simulink model "CM13_2024a_MachE_for_UA_HIL"  (R2024a)
settings: Solver=ode1  StartTime=0.0  StopTime=Inf  FixedStep=0.001  RelTol=1e-3  EnableMultiTasking=on
PreLoadFcn:
  | % if ~length(which('cmcmd')), cmenv; end
PostLoadFcn:
  | if any(exist('dsrtsu_mdlpostloadfcn', 'file') ~= 0), dsrtsu_mdlpostloadfcn('Execute', bdroot); end
InitFcn:
  | , if any(exist('rtifpga_mdlclblib', 'file') ~= 0), rtifpga_mdlclblib('Init', bdroot); end,
  | , if any(exist('dsmpb_private', 'file') ~= 0), dsmpb_private('dsmpb_mdlclblib', 'Init', bdroot); end,
values from neighbouring files (symbols this model uses):
  CoastDown =     [Run_Simulink.mat]
  limitedMCT =     [Run_Simulink.mat]
  MCT =     [Run_Simulink.mat]
  pMCT =     [Run_Simulink.mat]
  RealSimPara =     [Run_Simulink.mat]
  Ref_speed = [13 13.007895099 13.015778396 13.023649891 13.031509584 13.039357475 13.047193564 13.055017851 13.062830336 13.070631019 13.0784199 13.086196979 ... (2669 elements, 2669x1)]    [Ref_speed_and_time.mat]
  Ref_time = [0 0.01 0.02 0.03 0.04 0.05 0.06 0.07 0.08 0.09 0.1 0.11 ... (2669 elements, 2669x1)]    [Ref_speed_and_time.mat]
  US06 =     [Run_Simulink.mat]
undefined symbols (not defined in the file or in its folder): AccelCmd, ActTqLF_Nm_, ActTqLR_Nm_, ActTqRF_Nm_, ActTqRR_Nm_, BattChargeLimitMaxPwr, BattChargeLimitSocBpts, BattChargeLimitTbl, BattChrgCapcty, BattDischargeLimitSocBpts, BattDischargeLimitTbl, BattDischargeMaxPwr, BattNumCellsParallel, BattNumCellsSeries, BattOpenVoltCapBpts, BattOpenVoltTbl, BattResistSocBpts, BattResistTbl, BattResistTempBpts, BrakeMaxPrs, BrakeMaxTrq, ChassisDistCg2FrontAxle, ChassisDistCg2RearAxle, ChassisVehMass, CltchCmd, DecelCmd, DiffRatio, DiscIntNeverNeededParam, EnvGravCnst, EnvPrs, EnvTemp, FuelSpecificGrav, GearCmd, h, InitStates, lgSw, MtrEffSpdBpts, MtrEffTbl, MtrEffTrqBpts, MtrPwrMax, MtrTrqMax, planned_speed, planned_time, ref_speed, ref_time, rticanmm_blockfcn, rticanmm_initfcn, SteeringCmd, SupvsryCtrlRegenBrkCutOffTbl, SupvsryCtrlRegenSpdBpts, TestScnrioCycleNum, VEH
libraries: simulink x264, VSIGenLib x262, etargetslib x201, dsmpblib x161, CarMaker4SL x142, rtimmsu_dsrtlib x32, vehdynlibtire x24, autolibshared x19, vehdynlibsuspension x14, vehdynlibtirecommon x14, autolibutils x10, VsrLibWheel x8
(part 15 of 48)

== system CM13_2024a_MachE_for_UA_HIL/CarMaker/IPG Vehicle/Rototest and ORNL Interface/Format CM Powertrain Signals ==
  note: Can Bypass with my own brake model
  BrakingTorques : Inport
  RotoWheelSpd : Inport  Port=2
  AxlTrq : Inport  Port=3
  MaxRegen : Inport  Port=4
  Bus Creator1 : BusCreator  Inputs=42
  Bus Selector2 : BusSelector  OutputSignals=Brake IF Trq_WB FL,Brake IF Trq_WB FR,Brake IF Trq_WB RL,Brake IF Trq_WB RR
  BusCreator2 : BusCreator  Inputs=42
  Demux : Demux
  Demux1 : Demux  Outputs=42
      settings: DisplayOption=none
  Demux2 : Demux
  Discrete-Time Integrator{4..7} (4 alike) : DiscreteIntegrator  IntegratorMethod=Integration: Backward Euler  SampleTime=0.001  ICPrevOutput=DiscIntNeverNeededParam  ICPrevScaledInput=DiscIntNeverNeededParam
  Gain{5..8} (4 alike) : Gain  Gain=-1
  Ground{2..5} (4 alike) : Ground
  Ignition : Constant
  Memory{1..4} (4 alike) : Memory
  Operation Error : Constant  Value=4
  Operation State Driving : Constant  Value=4
  Product{1..4} (4 alike) : Product  RndMeth=Zero
  Saturation{1..4} (4 alike) : Saturate  UpperLimit=1  LowerLimit=-1
  Zero{1..5} (5 alike) : Constant  Value=0
  PowerTrainOutIdeal : Outport
  wires:
  Saturation4/1 -> Product4/2
  Demux1/3 -> BusCreator2/3  "PT IF OperationError"
  Demux1/2 -> BusCreator2/2  "PT IF OperationState"
  Demux1/40 -> BusCreator2/40  "PT IF WRR Trq_Supp2WC"
  Demux1/9 -> BusCreator2/9  "PT IF Trq_Supp2Bdy1B x"
  Discrete-Time Integrator6/1 -> Bus Creator1/29  "PT WRL rot"
  Demux1/1 -> BusCreator2/1  "PT IF Ignition"
  MaxRegen/1 -> Bus Creator1/28, Bus Creator1/21
  BusCreator2/1 -> PowerTrainOutIdeal/1
  Operation State Driving/1 -> Bus Creator1/2
  Gain8/1 -> Bus Creator1/38
  Demux1/16 -> BusCreator2/16  "PT IF WFL rotv"
  Demux1/21 -> BusCreator2/21  "PT IF WFL Trq_BrakeReg_max"
  Ground2/1 -> Bus Creator1/7
  Demux1/23 -> BusCreator2/23  "PT IF WFR rotv"
  Demux1/14 -> BusCreator2/14  "PT IF DL_iDiff_mean"
  Demux1/4 -> BusCreator2/4  "PT IF GearNo"
  Demux1/17 -> BusCreator2/17  "PT IF WFL Trq_B2W"
  Product3/1 -> Gain5/1
  Demux1/5 -> BusCreator2/5  "PT IF Engine_rotv"
  Demux1/11 -> BusCreator2/11  "PT IF Trq_Supp2Bdy1B z"
  Demux1/12 -> BusCreator2/12  "PT IF Trq_Supp2BdyEng x"
  Demux1/7 -> BusCreator2/7  "PT IF Trq_Supp2Bdy1 y"
  Discrete-Time Integrator5/1 -> Bus Creator1/22  "PT WFR rot"
  Demux1/42 -> BusCreator2/42  "PT IF WRR Trq_BrakeReg_max"
  Gain5/1 -> Bus Creator1/17
  Demux1/18 -> BusCreator2/18  "PT IF WFL Trq_Drive"
  Demux1/8 -> BusCreator2/8  "PT IF Trq_Supp2Bdy1 z"
  Demux1/38 -> BusCreator2/38  "PT IF WRR Trq_B2W"
  Memory4/1 -> Saturation4/1
  Demux1/10 -> BusCreator2/10  "PT IF Trq_Supp2Bdy1B y"
  Demux1/27 -> BusCreator2/27  "PT IF WFR Trq_BrakeReg"
  Demux1/24 -> BusCreator2/24  "PT IF WFR Trq_B2W"
  Demux1/25 -> BusCreator2/25  "PT IF WFR Trq_Drive"
  Demux1/26 -> BusCreator2/26  "PT IF WFR Trq_Supp2WC"
  Demux1/13 -> BusCreator2/13  "PT IF Trq_Supp2BdyEng y"
  Demux1/15 -> BusCreator2/15  "PT IF WFL rot"
  Bus Selector2/2 -> Product1/1  "<Brake IF Trq_WB FR>"
  Memory3/1 -> Saturation3/1
  Demux1/19 -> BusCreator2/19  "PT IF WFL Trq_Supp2WC"
  Demux1/22 -> BusCreator2/22  "PT IF WFR rot"
  Demux1/29 -> BusCreator2/29  "PT IF WRL rot"
  Demux1/33 -> BusCreator2/33  "PT IF WRL Trq_Supp2WC"
  Demux1/30 -> BusCreator2/30  "PT IF WRL rotv"
  Demux1/28 -> BusCreator2/28  "PT IF WFR Trq_BrakeReg_max"
  Demux1/35 -> BusCreator2/35  "PT IF WRL Trq_BrakeReg_max"
  Demux1/39 -> BusCreator2/39  "PT IF WRR Trq_Drive"
  Zero4/1 -> Bus Creator1/33, Bus Creator1/34, Bus Creator1/35
  Demux1/34 -> BusCreator2/34  "PT IF WRL Trq_BrakeReg"
  Demux1/37 -> BusCreator2/37  "PT IF WRR rotv"
  Demux1/31 -> BusCreator2/31  "PT IF WRL Trq_B2W"
  Demux1/32 -> BusCreator2/32  "PT IF WRL Trq_Drive"
  Demux1/36 -> BusCreator2/36  "PT IF WRR rot"
  Zero3/1 -> Bus Creator1/26, Bus Creator1/27
  Demux/4 -> Memory4/1, Discrete-Time Integrator7/1, Bus Creator1/37  "rotv RR"
  Zero2/1 -> Bus Creator1/19, Bus Creator1/20
  Zero1/1 -> Bus Creator1/5, Bus Creator1/4, Bus Creator1/12, Bus Creator1/14, Bus Creator1/13, Bus Creator1/11, Bus Creator1/10, Bus Creator1/9, Bus Creator1/8
  Demux1/20 -> BusCreator2/20  "PT IF WFL Trq_BrakeReg"
  Product2/1 -> Gain7/1
  Discrete-Time Integrator4/1 -> Bus Creator1/15  "PT WFL rot"
  Demux/2 -> Memory1/1, Discrete-Time Integrator5/1, Bus Creator1/23  "rotv FR"
  Discrete-Time Integrator7/1 -> Bus Creator1/36  "PtT WRR rot"
  Zero5/1 -> Bus Creator1/40, Bus Creator1/41, Bus Creator1/42
  Demux1/6 -> BusCreator2/6  "PT IF Trq_Supp2Bdy1 x"
  Demux1/41 -> BusCreator2/41  "PT IF WRR Trq_BrakeReg"
  BrakingTorques/1 -> Bus Selector2/1
  Operation Error/1 -> Bus Creator1/3
  Demux/3 -> Memory2/1, Discrete-Time Integrator6/1, Bus Creator1/30  "rotv RL"
  Memory1/1 -> Saturation1/1
  Ground4/1 -> Bus Creator1/6
  Bus Selector2/1 -> Product3/1  "<Brake IF Trq_WB FL>"
  Gain6/1 -> Bus Creator1/24
  Ignition/1 -> Bus Creator1/1  "PT Ignition"
  Memory2/1 -> Saturation2/1
  Saturation1/1 -> Product1/2
  Bus Selector2/3 -> Product2/1  "<Brake IF Trq_WB RL>"
  Gain7/1 -> Bus Creator1/31
  Demux/1 -> Memory3/1, Discrete-Time Integrator4/1, Bus Creator1/16  "rotv FL"
  Product4/1 -> Gain8/1
  Bus Creator1/1 -> Demux1/1
  Saturation2/1 -> Product2/2
  Product1/1 -> Gain6/1
  Bus Selector2/4 -> Product4/1  "<Brake IF Trq_WB RR>"
  Saturation3/1 -> Product3/2
  RotoWheelSpd/1 -> Demux/1
  AxlTrq/1 -> Demux2/1
  Demux2/1 -> Bus Creator1/18  "TrqDrv FL"
  Demux2/2 -> Bus Creator1/25  "TrqDrv FR"
  Demux2/3 -> Bus Creator1/32  "TrqDrv RL"
  Demux2/4 -> Bus Creator1/39  "TrqDrv RR"

== system CM13_2024a_MachE_for_UA_HIL/CarMaker/IPG Vehicle/Rototest and ORNL Interface/From Rototest ==
  Input : Inport
  Bus Creator : BusCreator  Inputs=30
  Bus Selector1 : BusSelector  OutputSignals=ActSpLF_rpm,ActSpRF_rpm,ActSpLR_rpm,ActSpRR_rpm
  Mux1 : Mux
  RotoTestEthRX : Subsystem  AncestorBlock=VSIGenLib/RotoTestEthRX
      mask Display:
      | color('white')
      | disp('RotTestEthTx')
      | port_label('output', 1, 'ID')
      | port_label('output', 2, 'ProtocolVer')
      | port_label('output', 3, 'ActTqLF (Nm)')
      | port_label('output', 4, 'RefRR_NmORrpm')
      | port_label('output', 5, 'ActTempLF (C)')
      | port_label('output', 6, 'ActTqRF (Nm)')
      | port_label('output', 7, 'ActSpRF (rpm)')
      | port_label('output', 8, 'ActTempRF (C)')
      | port_label('output', 9, 'ActTqLR (Nm)')
      | port_label('output', 10, 'ActSpLR (rpm)')
      | port_label('output', 11, 'ActTempLR (C)')
      | port_label('output', 12, 'ActTqRR (Nm)')
      | port_label('output', 13, 'ActSpRR (rpm)')
      | port_label('output', 14, 'ActTempRR (Nm)')
      | port_label('output', 15, 'RefLF (Nm)')
      | port_label('output', 16, 'RefRF (rpm)')
      | port_label('output', 17, 'RefLR (Nm)')
      | port_label('output', 18, 'RefRR (Nm)')
      | port_label('output', 19, 'UnitsStatusLF (enum)')
      | port_label('output', 20, 'UnitsStatusRF (enum)')
      | port_label('output', 21, 'UnitsStatusLR (enum)')
      | port_label('output', 22, 'UnitsStatusRR (enum)')
      | port_label('output', 23, 'WatchdogCnt (int)')
      | port_label('output', 24, 'FaultActive (enum)')
      | port_label('output', 25, 'WarningsActive (enum)')
      | port_label('output', 26, 'SpTqRR (enum)')
      | port_label('output', 27, 'SpTqLR (enum)')
      | port_label('output', 28, 'SpTqRF (enum)')
      | port_label('output', 29, 'SpTqLF (enum)')
      | port_label('output', 30, 'SystemActive (bool)')
  SpdAct : Outport
  AxlTrq : Outport  Port=2
  wires:
  RotoTestEthRX/8(ActTempRF_C) -> Bus Creator/8
  RotoTestEthRX/23(WatchdogCnt) -> Bus Creator/23
  RotoTestEthRX/18(RefRR_Nm) -> Bus Creator/18
  Mux1/1 -> SpdAct/1
  RotoTestEthRX/19(UnitsStatusLF) -> Bus Creator/19
  RotoTestEthRX/4(ActSpLF_rpm) -> Bus Creator/4
  Bus Creator/1 -> AxlTrq/1, Bus Selector1/1
  Bus Selector1/4 -> Mux1/4  "<ActSpRR_rpm>"
  RotoTestEthRX/24(FaultActive) -> Bus Creator/24
  RotoTestEthRX/22(UnitsStatusRR) -> Bus Creator/22
  Bus Selector1/3 -> Mux1/3  "<ActSpLR_rpm>"
  RotoTestEthRX/25(WarningsActive) -> Bus Creator/25
  Bus Selector1/1 -> Mux1/1  "<ActSpLF_rpm>"
  Bus Selector1/2 -> Mux1/2  "<ActSpRF_rpm>"
  RotoTestEthRX/5(ActTempLF_C) -> Bus Creator/5
  RotoTestEthRX/30(SystemActive) -> Bus Creator/30
  RotoTestEthRX/20(UnitsStatusRF) -> Bus Creator/20
  RotoTestEthRX/15(RefLF_Nm) -> Bus Creator/15
  RotoTestEthRX/16(RefRF_rpm) -> Bus Creator/16
  RotoTestEthRX/17(RefLR_Nm) -> Bus Creator/17
  RotoTestEthRX/2(ProtocolVer) -> Bus Creator/2
  RotoTestEthRX/7(ActSpRF_rpm) -> Bus Creator/7
  RotoTestEthRX/21(UnitsStatusLR) -> Bus Creator/21
  RotoTestEthRX/11(ActTempLR_C) -> Bus Creator/11
  RotoTestEthRX/1(ID) -> Bus Creator/1
  RotoTestEthRX/28(SpTqRF) -> Bus Creator/28
  RotoTestEthRX/29(SpTqLF) -> Bus Creator/29
  RotoTestEthRX/27(SpTqLR) -> Bus Creator/27
  RotoTestEthRX/26(SpTqRR) -> Bus Creator/26
  RotoTestEthRX/14(ActTempRR_Nm) -> Bus Creator/14
  RotoTestEthRX/3(ActTqLF_Nm) -> Bus Creator/3
  RotoTestEthRX/6(ActTqRF_Nm_) -> Bus Creator/6
  RotoTestEthRX/9(ActTqLR_Nm) -> Bus Creator/9
  RotoTestEthRX/13(ActSpRR_rpm) -> Bus Creator/13
  RotoTestEthRX/10(ActSpLR_rpm) -> Bus Creator/10
  RotoTestEthRX/12(ActTqRR_Nm) -> Bus Creator/12
  Input/1 -> RotoTestEthRX/1(Input)

== system CM13_2024a_MachE_for_UA_HIL/CarMaker/IPG Vehicle/Rototest and ORNL Interface/Get Wheel Spd Cmd Based on Wheel Dynamics ==
  BrakingTorques : Inport
  Trq_T2W : Inport  Port=2
  AxlTrq : Inport  Port=3
  MaxRegen : Inport  Port=4
  brkPressed : Inport  Port=5
  vehSpd : Inport  Port=6
  MATLAB Function : MATLAB Function  TreatAsAtomicUnit=on
  Saturation : Saturate  UpperLimit=100  LowerLimit=-100
  Saturation1 : Saturate  UpperLimit=300  LowerLimit=-300
  WheelSpdCmd : Subsystem  Commented=on
  Whl Dynamics & Format CM Powertrain Signal : Subsystem  Commented=on
  WhlSpdCmd : Outport
  tag scope: AxlTqrRotoTest=global
  wires:
  Whl Dynamics & Format CM Powertrain Signal/1(PowerTrainOutIdeal) -> WheelSpdCmd/1(In1)
  BrakingTorques/1 -> Whl Dynamics & Format CM Powertrain Signal/1(BrakingTorques)
  Trq_T2W/1 -> Whl Dynamics & Format CM Powertrain Signal/2(Trq_T2W)
  MaxRegen/1 -> Whl Dynamics & Format CM Powertrain Signal/4(MaxRegen)
  [SimOmega] -> MATLAB Function/1(u)
  Saturation/1 -> WhlSpdCmd/1
  AxlTrq/1 -> [AxlTqrRotoTest], Whl Dynamics & Format CM Powertrain Signal/3(AxlTrq)
  MATLAB Function/1(y) -> Saturation/1
  brkPressed/1 -> MATLAB Function/3(brkSw)
  vehSpd/1 -> MATLAB Function/2(vehSpd)

== system CM13_2024a_MachE_for_UA_HIL/CarMaker/IPG Vehicle/Rototest and ORNL Interface/RotoTrqPreprocess ==
  AxleTrqRaw : Inport
  Bus Selector1 : BusSelector  OutputSignals=ActTqLF_Nm_,ActTqRF_Nm_,ActTqLR_Nm_,ActTqRR_Nm
  Compare To Constant : simulink/Logic and Bit Operations/Compare To Constant  relop=>=  const=-15  OutDataTypeStr=boolean
  Compare To Constant1 : simulink/Logic and Bit Operations/Compare To Constant  relop=<=  const=0  OutDataTypeStr=boolean
  Data Type Conversion{1..4} (4 alike) : DataTypeConversion  OutDataTypeStr=double  SaturateOnIntegerOverflow=off  RndMeth=Floor
  FirstOrderFilterTau{,1..3} (4 alike) : VSIGenLib/FirstOrderFilterTau  SystemSampleTime=-1  VariantActivationTime=update diagram  AllowFlexibleInterface=on  Latency=0  AutoFrameSizeCalculation=off
  Ground : Ground
  Logical Operator : Logic  AllPortsSameDT=off  OutDataTypeStr=boolean
  ManualTrq_Nm : Constant  Value=0
  Mux : Mux
  Mux1 : Mux
  SatTrq : Saturate  UpperLimit=2800  LowerLimit=-2800
  Tau : Constant  Value=0.01
  TorqueIn : Switch  Criteria=u2 > Threshold  SaturateOnIntegerOverflow=off  InputSameDT=off
  "TorqueIn " : Switch  Criteria=u2 > Threshold  SaturateOnIntegerOverflow=off  InputSameDT=off
  AxleTrqRoto : Outport
  AxleTrqVeh : Outport  Port=2
  wires:
  Mux/1 -> AxleTrqRoto/1, TorqueIn/1
  ManualTrq_Nm/1 -> Mux1/4, Mux1/3, Mux1/2, Mux1/1
  Tau/1 -> FirstOrderFilterTau/2, FirstOrderFilterTau1/2, FirstOrderFilterTau2/2, FirstOrderFilterTau3/2
  Ground/1 -> "TorqueIn "/1
  Logical Operator/1 -> "TorqueIn "/2
  Data Type Conversion4/1 -> Mux/4  "RR"
  Data Type Conversion3/1 -> Mux/3  "LR"
  Mux1/1 -> TorqueIn/3
  [Switch] -> TorqueIn/2
  Bus Selector1/4 -> FirstOrderFilterTau3/1  "<ActTqRR_Nm>"
  Compare To Constant/1 -> Logical Operator/1
  Bus Selector1/3 -> FirstOrderFilterTau2/1  "<ActTqLR_Nm_>"
  Bus Selector1/2 -> FirstOrderFilterTau1/1  "<ActTqRF_Nm_>"
  TorqueIn/1 -> SatTrq/1
  "TorqueIn "/1 -> AxleTrqVeh/1  "Trq"
  FirstOrderFilterTau1/1 -> Data Type Conversion2/1
  Data Type Conversion2/1 -> Mux/2  "RF"
  AxleTrqRaw/1 -> Bus Selector1/1
  FirstOrderFilterTau/1 -> Data Type Conversion1/1
  FirstOrderFilterTau3/1 -> Data Type Conversion4/1
  Bus Selector1/1 -> FirstOrderFilterTau/1  "<ActTqLF_Nm_>"
  Compare To Constant1/1 -> Logical Operator/2
  SatTrq/1 -> "TorqueIn "/3, Compare To Constant1/1, Compare To Constant/1
  FirstOrderFilterTau2/1 -> Data Type Conversion3/1
  Data Type Conversion1/1 -> Mux/1  "LF"

== system CM13_2024a_MachE_for_UA_HIL/CarMaker/IPG Vehicle/Rototest and ORNL Interface/Subsystem2 ==
  AxlTorq : Inport
  BusCreator1 : BusCreator  Inputs=16
  BusCreator2 : BusCreator  Inputs=16
  Constant : Constant  Value=0
  Constant1 : Constant  Value=0
  Demux : Demux  Outputs=16
      settings: DisplayOption=none
  Terminator : Terminator
  Zero1 : Constant  Value=0
  Zero2 : Constant  Value=0
  Zero5 : Constant  Value=0
  BrakeUpd : Outport
  wires:
  Demux/9 -> BusCreator1/9  "Brake IF Trq_Reg_trg FL"
  Demux/6 -> BusCreator1/6  "Brake IF Trq_PB FR"
  Constant1/1 -> BusCreator2/1, BusCreator2/2  "Brake IF Trq_WB FL"
  Demux/14 -> BusCreator1/14  "Brake IF Trq_DriveSrc_trg d1"
  Zero2/1 -> BusCreator2/16, BusCreator2/15, BusCreator2/14, BusCreator2/13  "Brake IF Trq_DriveSrc_trg d3"
  Demux/11 -> BusCreator1/11  "Brake IF Trq_Reg_trg RL"
  Demux/15 -> BusCreator1/15  "Brake IF Trq_DriveSrc_trg d2"
  Demux/2 -> BusCreator1/2  "Brake IF Trq_WB FR"
  Demux/16 -> BusCreator1/16  "Brake IF Trq_DriveSrc_trg d3"
  Zero1/1 -> BusCreator2/12, BusCreator2/11, BusCreator2/10, BusCreator2/9  "Brake IF Trq_Reg_trg RR"
  Demux/4 -> BusCreator1/4  "Brake IF Trq_WB RR"
  Demux/3 -> BusCreator1/3  "Brake IF Trq_WB RL"
  Constant/1 -> BusCreator2/4, BusCreator2/3  "Brake IF Trq_WB RL"
  BusCreator1/1 -> BrakeUpd/1
  Demux/1 -> BusCreator1/1  "Brake IF Trq_WB FL"
  Demux/8 -> BusCreator1/8  "Brake IF Trq_PB RR"
  Demux/10 -> BusCreator1/10  "Brake IF Trq_Reg_trg FR"
  BusCreator2/1 -> Demux/1
  Demux/13 -> BusCreator1/13  "Brake IF Trq_DriveSrc_trg d0"
  Demux/5 -> BusCreator1/5  "Brake IF Trq_PB FL"
  Demux/7 -> BusCreator1/7  "Brake IF Trq_PB RL"
  Zero5/1 -> BusCreator2/8, BusCreator2/7, BusCreator2/6, BusCreator2/5  "Brake IF Trq_PB RR"
  Demux/12 -> BusCreator1/12  "Brake IF Trq_Reg_trg RR"
  AxlTorq/1 -> Terminator/1

== system CM13_2024a_MachE_for_UA_HIL/CarMaker/IPG Vehicle/Rototest and ORNL Interface/To Rototest with Band-Aid ==
  note: Torque Model: Low speed
      | Speed Model: Normal speed
  note: OutMode = 0 is Torque
      | OutMode = 1 is Speed
  note: Switch = 0 Overides
      | Switch = 1 Model
      | With Auto_MasterSW, User need to TurnOn_SW first
  SpeedCmd_rps : Inport
  AxleTrq_roto_Nm : Inport  Port=2
  BRAKE_PRESSED : Inport  Port=3
  Vehicle_Speed_kph : Inport  Port=4
  SpdAct : Inport  Port=5
  AND : Logic  Commented=on  IconShape=distinctive  AllPortsSameDT=off  OutDataTypeStr=boolean
  Auto_MasterSW : Subsystem  Commented=on
  Band-Aid : Subsystem
  Demux : Demux
  Demux1 : Demux
  Demux2 : Demux
  Logging : Subsystem  Commented=on
  MasterSw : Constant  Value=0
  Mode Override : Subsystem
  ModeOut : Switch  Criteria=u2 > Threshold  SaturateOnIntegerOverflow=off  InputSameDT=off
  ModeSwitch : MultiPortSwitch  DataPortOrder=Zero-based contiguous  Inputs=2  zeroidx=on  SaturateOnIntegerOverflow=off  InputSameDT=off
  Mux2 : Mux
  Mux4 : Mux
  Mux5 : Mux
  RateLimSpd : RateLimiter  RisingSlewLimit=500  FallingSlewLimit=-500  SampleTimeMode=inherited
  RotoTestEthTx : Subsystem  AncestorBlock=VSIGenLib/RotoTestEthTx
      mask Display:
      | color('white')
      | disp('RotTestEthTx')
      | port_label('input', 1, 'RefLF_NmORrpm')
      | port_label('input', 2, 'RefRF_NmORrpm')
      | port_label('input', 3, 'RefLR_NmORrpm')
      | port_label('input', 4, 'RefRR_NmORrpm')
      | port_label('input', 5, 'SqTrRR')
      | port_label('input', 6, 'SqTrLR')
      | port_label('input', 7, 'SqTrRF')
      | port_label('input', 8, 'SqTrLF')
      | port_label('input', 9, 'SystemActive')
      | port_label('output', 1, 'Status (bool)')
      | port_label('output', 2, 'Sent Bytes (int)')
  SatSpd : Saturate  UpperLimit=2000  LowerLimit=0
  SpeedOut : Switch  Criteria=u2 > Threshold  SaturateOnIntegerOverflow=off  InputSameDT=off
  SteeringSystem : Subsystem
  SystemActive : Constant  Value=0  OutDataTypeStr=uint8
  Terminator : Terminator  Commented=on
  Terminator1 : Terminator  Commented=on
  TrqSpd Override : Subsystem
  ZeroTorque : Constant  Value=0  OutDataTypeStr=uint8
  rads2rpm : Gain  Gain=9.5492965964254
  Out1 : Outport
  AutoMasterSW_Signal : Outport  Port=2
  tag scope: Switch=global
  wires:
  Mux4/1 -> ModeSwitch/2
  Demux/3 -> Mux2/3  "LRIn"
  Demux1/4 -> RotoTestEthTx/4(RefRR_NmORrpm)
  Demux/2 -> Mux2/2  "RFIn"
  MasterSw/1 -> AutoMasterSW_Signal/1, [Switch]
  TrqSpd Override/1(Ovr) -> SpeedOut/3
  ZeroTorque/1 -> Mux4/2, Mux4/3, Mux4/4, Mux4/1
  Demux/1 -> Mux2/1  "LFIn"
  SpeedOut/1 -> RateLimSpd/1
  RateLimSpd/1 -> SatSpd/1
  rads2rpm/1 -> Demux/1
  ModeSwitch/1 -> Demux1/1
  Demux/4 -> Mux2/4  "RRIn"
  Band-Aid/1(OutMode) -> Mux5/4, Mux5/3, Mux5/2, Mux5/1, ModeSwitch/1
  ModeOut/1 -> Demux2/1
  [Switch] -> SpeedOut/2
  SatSpd/1 -> ModeSwitch/3  "Spd"
  [Switch] -> ModeOut/2
  Mux5/1 -> ModeOut/1
  Demux2/1 -> RotoTestEthTx/5(SpTqRR)
  Demux1/3 -> RotoTestEthTx/3(RefLR_NmORrpm)
  Demux2/3 -> RotoTestEthTx/7(SpTqRF)
  Demux2/2 -> RotoTestEthTx/6(SpTqLR)
  SystemActive/1 -> RotoTestEthTx/9(SystemActive)
  RotoTestEthTx/1(Output) -> Out1/1  "ByteSend"
  Demux1/1 -> RotoTestEthTx/1(RefLF_NmORrpm)
  Demux1/2 -> RotoTestEthTx/2(RefRF_NmORrpm)
  Demux2/4 -> RotoTestEthTx/8(SpTqLF)
  SpeedCmd_rps/1 -> rads2rpm/1
  Mode Override/1(Ovr) -> ModeOut/3
  AxleTrq_roto_Nm/1 -> Band-Aid/2(InTrq_Nm)
  Mux2/1 -> Band-Aid/1(InSpd_rpm)
  Band-Aid/2(OutSpd_rpm) -> SpeedOut/1
  BRAKE_PRESSED/1 -> Band-Aid/3(BRAKE_PRESSED)
  Vehicle_Speed_kph/1 -> Band-Aid/4(VehSpd_kph)
  Auto_MasterSW/1(Auto_MasterSW) -> Terminator/1, AND/1  "AutoMasterSW_sig"
  AND/1 -> Terminator1/1  "MSW_sig"
  SpdAct/1 -> Auto_MasterSW/1(SpdAct)

== system CM13_2024a_MachE_for_UA_HIL/CarMaker/IPG Vehicle/SUMO Spd/dSPACE TCP Out ==
  ByteSend : Inport
  nMsgSend : Inport  Port=2
  sendTrigger : Inport  Port=3
  Constant1 : Constant  Value=0
  Data Type Conversion4 : DataTypeConversion  SaturateOnIntegerOverflow=off  RndMeth=Floor
  Display7 : Display
  Transmit_Out [TCP Ref Speed]1 : dsmpblib/Data Outport  Priority=-10000
      settings: SourceProductName=dSPACE Model Interface Package for Simulink (MIPS)
  switch for 0.1 send out : Switch  Criteria=u2 > Threshold  SaturateOnIntegerOverflow=off  InputSameDT=off
  wires:
  Constant1/1 -> switch for 0.1 send out/3
  nMsgSend/1 -> Data Type Conversion4/1
  Data Type Conversion4/1 -> switch for 0.1 send out/1, Display7/1
  switch for 0.1 send out/1 -> Transmit_Out [TCP Ref Speed]1/2  "sendByteSize_RealSimPack"
  ByteSend/1 -> Transmit_Out [TCP Ref Speed]1/1
  sendTrigger/1 -> switch for 0.1 send out/2

== system CM13_2024a_MachE_for_UA_HIL/CarMaker/IPG Vehicle/Steering Angle HIL/Steering Override ==
  note: IPG
      | 	positive left turn, negative right turn
  note: SteerOverrideSwitch
      | 0: use IPG steer
      | 1: use CAN steer
      | 2: use manual input
  SteerAngCAN_in : Inport
  <VhclCtrl Steering Ang> : Inport  Port=2
  Gain : Gain
  Gain1 : Gain  Gain=pi/180
  Multiport Switch : MultiPortSwitch  DataPortOrder=Zero-based contiguous  zeroidx=on  SaturateOnIntegerOverflow=off  InputSameDT=off
  SteerManual : Constant  Value=0
  SteerOverrideSwitch : Constant  Value=0
  VhclCtrl Steering Ang : Outport
  wires:
  SteerManual/1 -> Gain/1
  Gain1/1 -> Multiport Switch/3  "SteerAngCAN_rad"
  Gain/1 -> Multiport Switch/4
  SteerOverrideSwitch/1 -> Multiport Switch/1
  Multiport Switch/1 -> VhclCtrl Steering Ang/1  "VhclCtrl Steering Ang"
  <VhclCtrl Steering Ang>/1 -> Multiport Switch/2
  SteerAngCAN_in/1 -> Gain1/1

== system CM13_2024a_MachE_for_UA_HIL/CarMaker_new/IPG Vehicle/AEB Flag/RTICANMM ControllerSetup ==
  VariationInput : Inport
  Reset : Inport  Port=2
  DSRT Data Hook : rtimmsu_dsrtlib/Data Hook  ControllerName=MachE_FD1  PortID=RTICANMMMachE_FD1  BlockSet=RTICANMM  blockdata=struct('version','1.0')  MMType=ControllerSetup
  ModelClose : Subsystem  mask(RTICANMMModelClose){}
  RTICANMMCHANNEL_TLC : S-Function  FunctionName=rticanmm_tlc_adv  Parameters='DSRT',-1,-1,-1,500,26711143421  SFunctionDeploymentMode=off  EnableBusSupport=off  mask(RTICANMMCHANNEL_TLC){}
  Variation_DTC : DataTypeConversion
  sfcn : S-Function  InitFcn=rticanmm_initfcn(gcb, 'SFCNs')  FunctionName=RTICANMM_SETUP_MachE_FD1  SFunctionDeploymentMode=off  EnableBusSupport=off
      mask init:
      | rticanmm_initfcn(gcb, 'SFCNs')
  BUS_STATE : Outport
  STATUS_BIT0_ERROR : Outport  Port=2
  STATUS_BIT1_ERROR : Outport  Port=3
  STATUS_CRC_ERROR : Outport  Port=4
  wires:
  Reset/1 -> sfcn/2
  sfcn/1 -> BUS_STATE/1
  sfcn/2 -> STATUS_BIT0_ERROR/1
  sfcn/3 -> STATUS_BIT1_ERROR/1
  sfcn/4 -> STATUS_CRC_ERROR/1
  VariationInput/1 -> Variation_DTC/1
  Variation_DTC/1 -> sfcn/1

== system CM13_2024a_MachE_for_UA_HIL/CarMaker_new/IPG Vehicle/AEB Flag/RTICANMM MainBlock ==
  DSRT Data Hook : rtimmsu_dsrtlib/Data Hook  ControllerName=MachE_FD1  PortID=RTICANMMMachE_FD1  BlockSet=RTICANMM  blockdata=struct('version','1.0')  Variant=MachE_FD1  MMType=mainsetup
  ModelClose : Subsystem  mask(RTICANMMModelClose){}
  TRC Exclusion : rtimmsu_dsrtlib/TRC Exclusion
  converter : Subsystem  mask(CANnedyVector2Bus){}
      mask help: Do not change.
      mask Display: disp('Vector to\nBus')
  sfcn : S-Function  InitFcn=rticanmm_initfcn(gcb, 'SFCNs')  FunctionName=RTICANMM_MAIN_MachE_FD1  SFunctionDeploymentMode=off  EnableBusSupport=off
      mask init:
      | rticanmm_initfcn(gcb, 'SFCNs')
  RX_Data : Outport
  wires:
  converter/1(out) -> RX_Data/1
  sfcn/1 -> converter/1(in_1)
  sfcn/2 -> converter/2(in_2)
  sfcn/3 -> converter/3(in_3)
  sfcn/4 -> converter/4(in_4)
  sfcn/5 -> converter/5(in_5)
  sfcn/6 -> converter/6(in_6)
  sfcn/7 -> converter/7(in_7)

== system CM13_2024a_MachE_for_UA_HIL/CarMaker_new/IPG Vehicle/Actuation and Outputs/MOOG Brake Actuator ==
  Brake Pedal command [%] : Inport
  " CAN Settings" : Subsystem
  BrakePedal Target Position Manual Bypass : Constant  Value=0
  BrakePedal TargetPosition Bypass Enable : Constant  Value=0
  Bus Selector : BusSelector  OutputSignals=ControlWord,TargetPositionFinal_cnt
  ControlWord bypass Enable : Constant  Value=0
  ControlWord bypass Override value : Constant  Value=0
  Data Type Conversion : DataTypeConversion  SaturateOnIntegerOverflow=off  RndMeth=Floor
  Data Type Conversion1 : DataTypeConversion  SaturateOnIntegerOverflow=off  RndMeth=Floor
  Data Type Conversion2 : DataTypeConversion  SaturateOnIntegerOverflow=off  RndMeth=Floor
  Gain : Gain
  Gain1 : Gain
  MOOG Interface : Subsystem
  RPDO3\ControlWord0\ISignal Value\ControlWord0 Value [BrakeAct_Config\Simulated ECUs\CANOpen_MOOG_02\Controller\TX\PDUs] : dsmpblib/Data Outport  Priority=-10000
      settings: SourceProductName=dSPACE Model Interface Package for Simulink (MIPS)
  RPDO3\ModesOfOperation\ISignal Value\ModesOfOperation Value [BrakeAct_Config\Simulated ECUs\CANOpen_MOOG_02\Controller\TX\PDUs] : dsmpblib/Data Outport  Priority=-10000
      settings: SourceProductName=dSPACE Model Interface Package for Simulink (MIPS)
  RPDO3\TargetPosition\ISignal Value\TargetPosition Value [BrakeAct_Config\Simulated ECUs\CANOpen_MOOG_02\Controller\TX\PDUs] : dsmpblib/Data Outport  Priority=-10000
      settings: SourceProductName=dSPACE Model Interface Package for Simulink (MIPS)
  Rate Limiter : RateLimiter  RisingSlewLimit=50  FallingSlewLimit=-50  SampleTimeMode=inherited
  Sine Wave : Sin  Amplitude=50  Bias=50  SampleTime=0
  Switch : Switch  Criteria=u2 > Threshold  SaturateOnIntegerOverflow=off  InputSameDT=off
  Switch1 : Switch  Criteria=u2 > Threshold  SaturateOnIntegerOverflow=off  InputSameDT=off
  Switch2 : Switch  Criteria=u2 > Threshold  SaturateOnIntegerOverflow=off  InputSameDT=off
  TPDO3\ActualPosition\ISignal Value\ActualPosition Value [BrakeAct_Config\Simulated ECUs\CANOpen_MOOG_02\Controller\RX\PDUs] : dsmpblib/Data Inport  Priority=10000
      settings: SourceProductName=dSPACE Model Interface Package for Simulink (MIPS)
  TPDO3\ModesOfOperationDisplay\ISignal Value\ModesOfOperationDisplay Value [BrakeAct_Config\Simulated ECUs\CANOpen_MOOG_02\Controller\RX\PDUs] : dsmpblib/Data Inport  Priority=10000
      settings: SourceProductName=dSPACE Model Interface Package for Simulink (MIPS)
  TPDO3\StatusWord0\ISignal Value\StatusWord0 Value [BrakeAct_Config\Simulated ECUs\CANOpen_MOOG_02\Controller\RX\PDUs] : dsmpblib/Data Inport  Priority=10000
      settings: SourceProductName=dSPACE Model Interface Package for Simulink (MIPS)
  Terminator : Terminator
  Terminator1 : Terminator
  Terminator2 : Terminator
  constant : Constant
  trace selection : Constant  Value=0
  wires:
  Switch/1 -> Switch2/1
  MOOG Interface/1(Commands) -> Bus Selector/1
  MOOG Interface/2(ActualPosition [pct]) -> Terminator/1  "BrakePedal_ActualPosition_pct"
  Bus Selector/2 -> Data Type Conversion2/1  "<TargetPositionFinal_cnt>"
  MOOG Interface/3(BrakeActuatorReady) -> Terminator1/1  "BrakeActuator_Ready_bool"
  Sine Wave/1 -> Switch/1
  Data Type Conversion2/1 -> RPDO3\TargetPosition\ISignal Value\TargetPosition Value [BrakeAct_Config\Simulated ECUs\CANOpen_MOOG_02\Controller\TX\PDUs]/1, Gain1/1  "TargetPosition_Cnt_Final"
  constant/1 -> Data Type Conversion/1
  BrakePedal TargetPosition Bypass Enable/1 -> Switch2/2
  trace selection/1 -> Switch/2
  TPDO3\ModesOfOperationDisplay\ISignal Value\ModesOfOperationDisplay Value [BrakeAct_Config\Simulated ECUs\CANOpen_MOOG_02\Controller\RX\PDUs]/1 -> MOOG Interface/5(Mode of operation in)  "Modes of operations"
  Data Type Conversion1/1 -> RPDO3\ControlWord0\ISignal Value\ControlWord0 Value [BrakeAct_Config\Simulated ECUs\CANOpen_MOOG_02\Controller\TX\PDUs]/1  "ControlWord_Final"
  Gain/1 -> MOOG Interface/2(TargetPosition [pct])  "BrakePedal_TargetlPosition_pct"
  Switch1/1 -> Data Type Conversion1/1
  TPDO3\ActualPosition\ISignal Value\ActualPosition Value [BrakeAct_Config\Simulated ECUs\CANOpen_MOOG_02\Controller\RX\PDUs]/1 -> MOOG Interface/4(ActualPosition_cnt in)  "ActualPosition_cnt"
  Bus Selector/1 -> Switch1/3  "<ControlWord>"
  ControlWord bypass Override value/1 -> Switch1/1
  TPDO3\StatusWord0\ISignal Value\StatusWord0 Value [BrakeAct_Config\Simulated ECUs\CANOpen_MOOG_02\Controller\RX\PDUs]/1 -> MOOG Interface/3(StatusWord in)  "StatusWord0"
  BrakePedal Target Position Manual Bypass/1 -> Rate Limiter/1
  ControlWord bypass Enable/1 -> Switch1/2
  Brake Pedal command [%]/1 -> Switch2/3
  " CAN Settings"/1(CAN_CommsOK_Flg) -> MOOG Interface/1(CAN_CommsOK_Flg)
  Gain1/1 -> Terminator2/1  "BrakePedal_CmdFinal_pct"
  Rate Limiter/1 -> Switch/3
  Switch2/1 -> Gain/1
  Data Type Conversion/1 -> RPDO3\ModesOfOperation\ISignal Value\ModesOfOperation Value [BrakeAct_Config\Simulated ECUs\CANOpen_MOOG_02\Controller\TX\PDUs]/1

== system CM13_2024a_MachE_for_UA_HIL/CarMaker_new/IPG Vehicle/Actuation and Outputs/Vehicle Accel Pedal Voltage Output ==
  note: Default value for MachE:
      | APP1_CmdFinal_V: 0.8016
      | APP2_CmdFinal_V: 0.4008
  APP_pct : Inport
  APP1Tbl : Lookup_n-D  NumberOfTableDimensions=1  BreakpointsForDimension1=[0 100]  Table=[16 78.8]  InternalRulePriority=Speed  RndMeth=Simplest
  APP2Tbl : Lookup_n-D  NumberOfTableDimensions=1  BreakpointsForDimension1=[0 100]  Table=[8 39.4]  InternalRulePriority=Speed  RndMeth=Simplest
  AccelPosition Bypass Enable : Constant  Value=0
  AccelPosition Manual Bypass [%] : Constant  Value=0
  Gain : Gain
  Gain1 : Gain
  Gain2 : Gain
  Gain3 : Gain  Gain=1/100
  Gain4 : Gain  Gain=1/100
  Product2 : Product
  Product3 : Product
  Rate Limiter : RateLimiter  RisingSlewLimit=50  FallingSlewLimit=-50  SampleTimeMode=inherited
  Switch2 : Switch  Criteria=u2 > Threshold  SaturateOnIntegerOverflow=off  InputSameDT=off
  TPS Channel 1 : dsmpblib/Data Outport  Priority=-10000
      settings: SourceProductName=dSPACE Model Interface Package for Simulink (MIPS)
  TPS Channel 2 : dsmpblib/Data Outport  Priority=-10000
      settings: SourceProductName=dSPACE Model Interface Package for Simulink (MIPS)
  Terminator2 : Terminator
  VRef : Constant  Value=5.01
  wires:
  Switch2/1 -> APP1Tbl/1, APP2Tbl/1, Gain2/1  "APP_CmdFinal_pct"
  APP_pct/1 -> Switch2/3
  AccelPosition Manual Bypass [%]/1 -> Rate Limiter/1
  AccelPosition Bypass Enable/1 -> Switch2/2
  Gain/1 -> TPS Channel 2/1  "APP2_CmdFinal_V"
  Gain1/1 -> TPS Channel 1/1  "APP1_CmdFinal_V"
  Gain2/1 -> Terminator2/1  "AccelPedal_CmdFinal_pct"
  Rate Limiter/1 -> Switch2/1
  VRef/1 -> Product2/2, Product3/1
  Gain4/1 -> Product3/2
  Product2/1 -> Gain1/1
  APP2Tbl/1 -> Gain4/1
  Gain3/1 -> Product2/1
  Product3/1 -> Gain/1
  APP1Tbl/1 -> Gain3/1

== system CM13_2024a_MachE_for_UA_HIL/CarMaker_new/IPG Vehicle/Brake/CreateBus Vhcl.Wheel.PT ==
  In : Inport
  BusCreator1 : BusCreator  Inputs=20
  Demux1 : Demux  Outputs=20
      settings: DisplayOption=none
  Out : Outport  VectorParamsAs1DForOutWhenUnconnected=off
  wires:
  Demux1/20 -> BusCreator1/20  "Vhcl Trq_DriveSrc_trg d3"
  Demux1/19 -> BusCreator1/19  "Vhcl Trq_DriveSrc_trg d2"
  Demux1/18 -> BusCreator1/18  "Vhcl Trq_DriveSrc_trg d1"
  Demux1/17 -> BusCreator1/17  "Vhcl Trq_DriveSrc_trg d0"
  Demux1/16 -> BusCreator1/16  "Vhcl Wheel RR WhlBearing"
  Demux1/15 -> BusCreator1/15  "Vhcl Wheel RR Trq_T2W"
  Demux1/14 -> BusCreator1/14  "Vhcl Wheel RR Trq_BrakeReg_trg"
  Demux1/13 -> BusCreator1/13  "Vhcl Wheel RR Trq_Brake"
  Demux1/12 -> BusCreator1/12  "Vhcl Wheel RL WhlBearing"
  Demux1/11 -> BusCreator1/11  "Vhcl Wheel RL Trq_T2W"
  Demux1/10 -> BusCreator1/10  "Vhcl Wheel RL Trq_BrakeReg_trg"
  Demux1/9 -> BusCreator1/9  "Vhcl Wheel RL Trq_Brake"
  Demux1/8 -> BusCreator1/8  "Vhcl Wheel FR WhlBearing"
  Demux1/7 -> BusCreator1/7  "Vhcl Wheel FR Trq_T2W"
  Demux1/6 -> BusCreator1/6  "Vhcl Wheel FR Trq_BrakeReg_trg"
  Demux1/5 -> BusCreator1/5  "Vhcl Wheel FR Trq_Brake"
  Demux1/4 -> BusCreator1/4  "Vhcl Wheel FL WhlBearing"
  Demux1/3 -> BusCreator1/3  "Vhcl Wheel FL Trq_T2W"
  Demux1/2 -> BusCreator1/2  "Vhcl Wheel FL Trq_BrakeReg_trg"
  Demux1/1 -> BusCreator1/1  "Vhcl Wheel FL Trq_Brake"
  BusCreator1/1 -> Out/1
  In/1 -> Demux1/1

== system CM13_2024a_MachE_for_UA_HIL/CarMaker_new/IPG Vehicle/CarAndTrailer/CarAndTrailerUpd ==
  Sync_In : Inport
  Vhcl.Steering : Inport  Port=2
  Vhcl.Motion : Inport  Port=3
  Vhcl.PoI : Inport  Port=4
  Vhcl.Wheel.FL : Inport  Port=5
  Vhcl.Wheel.FR : Inport  Port=6
  Vhcl.Wheel.RL : Inport  Port=7
  Vhcl.Wheel.RR : Inport  Port=8
  Car.Hitch.FrcTrq : Inport  Port=9
  Vhcl.Fr1A : Inport  Port=10
  CarAndTrailerUpd : S-Function  FunctionName=CM_Sfun  Parameters='CarAndTrUpd'  SFunctionDeploymentMode=off  EnableBusSupport=off
  CreateBus Brake.IF.In : Subsystem
  Sync_Out : Outport  VectorParamsAs1DForOutWhenUnconnected=off
  Brake.IF.In : Outport  Port=2  VectorParamsAs1DForOutWhenUnconnected=off
  wires:
  Vhcl.Fr1A/1 -> CarAndTrailerUpd/10  "user vehicle only"
  Vhcl.Steering/1 -> CarAndTrailerUpd/2
  Vhcl.Motion/1 -> CarAndTrailerUpd/3
  Vhcl.PoI/1 -> CarAndTrailerUpd/4
  Vhcl.Wheel.FL/1 -> CarAndTrailerUpd/5
  Vhcl.Wheel.FR/1 -> CarAndTrailerUpd/6
  Car.Hitch.FrcTrq/1 -> CarAndTrailerUpd/9
  Vhcl.Wheel.RR/1 -> CarAndTrailerUpd/8
  Vhcl.Wheel.RL/1 -> CarAndTrailerUpd/7
  CarAndTrailerUpd/2 -> CreateBus Brake.IF.In/1(In)
  CreateBus Brake.IF.In/1(Out) -> Brake.IF.In/1
  CarAndTrailerUpd/1 -> Sync_Out/1
  Sync_In/1 -> CarAndTrailerUpd/1

== system CM13_2024a_MachE_for_UA_HIL/CarMaker_new/IPG Vehicle/CarAndTrailer/Forces ==
  Sync_In : Inport
  TireFL_In : Inport  Port=2
  TireFR_In : Inport  Port=3
  TireRL_In : Inport  Port=4
  TireRR_In : Inport  Port=5
  lSpring : Inport  Port=6
  vDamp : Inport  Port=7
  lStabi : Inport  Port=8
  lBuf : Inport  Port=9
  External Suspension Forces : Subsystem
  Suspension Forces : Subsystem
  Tires : Subsystem
  Vehicle Forces : Subsystem
  Sync_Out : Outport  VectorParamsAs1DForOutWhenUnconnected=off
  Car.Virtual : Outport  Port=2  VectorParamsAs1DForOutWhenUnconnected=off
  Car.Aero : Outport  Port=3  VectorParamsAs1DForOutWhenUnconnected=off
  Car.Load : Outport  Port=4  VectorParamsAs1DForOutWhenUnconnected=off
  TireFL_Out : Outport  Port=5  VectorParamsAs1DForOutWhenUnconnected=off
  TireFR_Out : Outport  Port=6  VectorParamsAs1DForOutWhenUnconnected=off
  TireRL_Out : Outport  Port=7  VectorParamsAs1DForOutWhenUnconnected=off
  TireRR_Out : Outport  Port=8  VectorParamsAs1DForOutWhenUnconnected=off
  FSpring_ext : Outport  Port=9  VectorParamsAs1DForOutWhenUnconnected=off
  FDamp_ext : Outport  Port=10  VectorParamsAs1DForOutWhenUnconnected=off
  FStabi_ext : Outport  Port=11  VectorParamsAs1DForOutWhenUnconnected=off
  FBuf_ext : Outport  Port=12  VectorParamsAs1DForOutWhenUnconnected=off
  wires:
  lBuf/1 -> External Suspension Forces/5(lBuf), Suspension Forces/5(lBuf)
  lStabi/1 -> External Suspension Forces/4(lStabi), Suspension Forces/4(lStabi)
  vDamp/1 -> External Suspension Forces/3(vDamp), Suspension Forces/3(vDamp)
  Tires/4(TireRR_Out) -> TireRR_Out/1
  Tires/3(TireRL_Out) -> TireRL_Out/1
  Tires/2(TireFR_Out) -> TireFR_Out/1
  Tires/1(TireFL_Out) -> TireFL_Out/1
  TireRR_In/1 -> Tires/5(TireRR_In)
  TireRL_In/1 -> Tires/4(TireRL_In)
  TireFR_In/1 -> Tires/3(TireFR_In)
  TireFL_In/1 -> Tires/2(TireFL_In)
  External Suspension Forces/4(FBuf_ext) -> FBuf_ext/1
  Sync_In/1 -> External Suspension Forces/1(Sync_In), Tires/1(Sync_In), Vehicle Forces/1(Sync_In)
  Vehicle Forces/1(Sync_Out) -> Suspension Forces/1(Sync_In)
  Vehicle Forces/2(Car.Virtual) -> Car.Virtual/1
  Vehicle Forces/3(Car.Aero) -> Car.Aero/1
  Vehicle Forces/4(Car.Load) -> Car.Load/1
  lSpring/1 -> External Suspension Forces/2(lSpring), Suspension Forces/2(lSpring)
  External Suspension Forces/2(FDamp_ext) -> FDamp_ext/1
  External Suspension Forces/3(FStabi_ext) -> FStabi_ext/1
  External Suspension Forces/1(FSpring_ext) -> FSpring_ext/1
  Suspension Forces/1(Sync_Out) -> Sync_Out/1

== system CM13_2024a_MachE_for_UA_HIL/CarMaker_new/IPG Vehicle/CarAndTrailer/Kinematics ==
  Sync_In : Inport
  Steer.IF : Inport  Port=2
  Kinematics : S-Function  FunctionName=CM_Sfun  Parameters='Kinematics'  SFunctionDeploymentMode=off  EnableBusSupport=off
  Sync_Out : Outport  VectorParamsAs1DForOutWhenUnconnected=off
  TireFL_In : Outport  Port=2  VectorParamsAs1DForOutWhenUnconnected=off
  TireFR_In : Outport  Port=3  VectorParamsAs1DForOutWhenUnconnected=off
  TireRL_In : Outport  Port=4  VectorParamsAs1DForOutWhenUnconnected=off
  TireRR_In : Outport  Port=5  VectorParamsAs1DForOutWhenUnconnected=off
  lSpring : Outport  Port=6  VectorParamsAs1DForOutWhenUnconnected=off
  vDamp : Outport  Port=7  VectorParamsAs1DForOutWhenUnconnected=off
  lStabi : Outport  Port=8  VectorParamsAs1DForOutWhenUnconnected=off
  lBuf : Outport  Port=9  VectorParamsAs1DForOutWhenUnconnected=off
  wires:
  Kinematics/9 -> lBuf/1
  Kinematics/8 -> lStabi/1
  Kinematics/2 -> TireFL_In/1
  Kinematics/3 -> TireFR_In/1
  Kinematics/4 -> TireRL_In/1
  Kinematics/5 -> TireRR_In/1
  Kinematics/6 -> lSpring/1
  Kinematics/7 -> vDamp/1
  Sync_In/1 -> Kinematics/1
  Kinematics/1 -> Sync_Out/1
  Steer.IF/1 -> Kinematics/2

== system CM13_2024a_MachE_for_UA_HIL/CarMaker_new/IPG Vehicle/CarAndTrailer/Kinetics ==
  Sync_In : Inport
  Car.Virtual : Inport  Port=2
  Car.Aero : Inport  Port=3
  Car.Load : Inport  Port=4
  TireFL.Out : Inport  Port=5
  TireFR.Out : Inport  Port=6
  TireRL.Out : Inport  Port=7
  TireRR.Out : Inport  Port=8
  FSpring_ext : Inport  Port=9
  FDamp_ext : Inport  Port=10
  FStabi_ext : Inport  Port=11
  FBuf_ext : Inport  Port=12
  Bus Creator : BusCreator  Inputs=4
  Bus Creator1 : BusCreator  Inputs=12
  Bus Creator2 : BusCreator  Inputs=6
  Bus Creator3 : BusCreator  Inputs=6
  Bus Creator4 : BusCreator  Inputs=4
  Demux : Demux  Outputs=12
      settings: DisplayOption=none
  Demux1 : Demux  Outputs=6
      settings: DisplayOption=none
  Demux2 : Demux  Outputs=6
      settings: DisplayOption=none
  Demux3 : Demux
      settings: DisplayOption=none
  Demux4 : Demux
      settings: DisplayOption=none
  Kinetics : S-Function  FunctionName=CM_Sfun  Parameters='Kinetics'  SFunctionDeploymentMode=off  EnableBusSupport=off
  Sync_Out : Outport  VectorParamsAs1DForOutWhenUnconnected=off
  Trailer.Load : Outport  Port=2  VectorParamsAs1DForOutWhenUnconnected=off
  Car.Hitch : Outport  Port=3  VectorParamsAs1DForOutWhenUnconnected=off
  Car.Fr1 : Outport  Port=4  VectorParamsAs1DForOutWhenUnconnected=off
  Car.Trq_T2W : Outport  Port=5  VectorParamsAs1DForOutWhenUnconnected=off
  WheelCarrier.Misc : Outport  Port=6  VectorParamsAs1DForOutWhenUnconnected=off
  wires:
  FBuf_ext/1 -> Kinetics/12
  Sync_In/1 -> Kinetics/1
  Kinetics/1 -> Sync_Out/1
  Car.Aero/1 -> Kinetics/3
  Car.Virtual/1 -> Kinetics/2
  Bus Creator1/1 -> Trailer.Load/1
  Demux/1 -> Bus Creator1/1  "Trailer Load_0 mass"
  Demux/2 -> Bus Creator1/2  "Trailer Load_0 tx"
  Demux/3 -> Bus Creator1/3  "Trailer Load_0 ty"
  Demux/4 -> Bus Creator1/4  "Trailer Load_0 tz"
  Kinetics/2 -> Demux/1
  Demux/5 -> Bus Creator1/5  "Trailer Load_1 mass"
  Demux/6 -> Bus Creator1/6  "Trailer Load_1 tx"
  Demux/7 -> Bus Creator1/7  "Trailer Load_1 ty"
  Demux/8 -> Bus Creator1/8  "Trailer Load_1 tz"
  Demux/9 -> Bus Creator1/9  "Trailer Load_2 mass"
  Demux/10 -> Bus Creator1/10  "Trailer Load_2 tx"
  Demux/11 -> Bus Creator1/11  "Trailer Load_2 ty"
  Demux/12 -> Bus Creator1/12  "Trailer Load_2 tz"
  Demux1/1 -> Bus Creator2/1  "Car Hitch tx"
  Demux1/2 -> Bus Creator2/2  "Car Hitch ty"
  Demux1/3 -> Bus Creator2/3  "Car Hitch tz"
  Demux1/4 -> Bus Creator2/4  "Car Hitch vx"
  Demux1/5 -> Bus Creator2/5  "Car Hitch vy"
  Demux1/6 -> Bus Creator2/6  "Car Hitch vz"
  Kinetics/3 -> Demux1/1
  Bus Creator2/1 -> Car.Hitch/1
  Demux2/1 -> Bus Creator3/1  "Car Fr1 rx"
  Demux2/2 -> Bus Creator3/2  "Car Fr1 ry"
  Demux2/3 -> Bus Creator3/3  "Car Fr1 rz"
  Demux2/4 -> Bus Creator3/4  "Car Fr1 rvx"
  Demux2/5 -> Bus Creator3/5  "Car Fr1 rvy"
  Demux2/6 -> Bus Creator3/6  "Car Fr1 rvz"
  Bus Creator3/1 -> Car.Fr1/1
  Kinetics/4 -> Demux2/1
  Car.Load/1 -> Kinetics/4
  Demux3/1 -> Bus Creator4/1  "car Susp FL GenInert2"
  Demux3/2 -> Bus Creator4/2  "car Susp FR GenInert2"
  Demux3/3 -> Bus Creator4/3  "car Susp FL GenFrc2"
  Demux3/4 -> Bus Creator4/4  "car Susp FR GenFrc2"
  Bus Creator4/1 -> WheelCarrier.Misc/1
  Bus Creator/1 -> Car.Trq_T2W/1
  Demux4/4 -> Bus Creator/4  "Car Trq_T2WRR"
  Demux4/3 -> Bus Creator/3  "Car Trq_T2WRL"
  Demux4/2 -> Bus Creator/2  "Car Trq_T2WFR"
  Demux4/1 -> Bus Creator/1  "Car Trq_T2WFL"
  TireFL.Out/1 -> Kinetics/5
  TireFR.Out/1 -> Kinetics/6
  TireRL.Out/1 -> Kinetics/7
  TireRR.Out/1 -> Kinetics/8
  FSpring_ext/1 -> Kinetics/9
  FDamp_ext/1 -> Kinetics/10
  FStabi_ext/1 -> Kinetics/11
  Kinetics/6 -> Demux3/1
  Kinetics/5 -> Demux4/1

== system CM13_2024a_MachE_for_UA_HIL/CarMaker_new/IPG Vehicle/CarAndTrailer/Steering ==
  note: When replacing the entire steering system,
      | be sure to disable the IPG steering model by using the steering
      | model 'Model Manager off' in the vehicle GUI.
  Sync_In : Inport
  VhclCtrl.Steering : Inport  Port=2
  Bus Creator1 : BusCreator  Inputs=16
  Bus Creator2 : BusCreator  Inputs=5
  Demux : Demux  Outputs=21
      settings: DisplayOption=none
  Steering : S-Function  FunctionName=CM_Sfun  Parameters='Steering'  SFunctionDeploymentMode=off  EnableBusSupport=off
  Terminator : Terminator
  Sync_Out : Outport  VectorParamsAs1DForOutWhenUnconnected=off
  Steer.IF : Outport  Port=2  VectorParamsAs1DForOutWhenUnconnected=off
  wires:
  Demux/21 -> Bus Creator2/5  "Steering IF R Inert"
  Demux/20 -> Bus Creator2/4  "Steering IF R Frc"
  Demux/19 -> Bus Creator2/3  "Steering IF L Inert"
  Demux/18 -> Bus Creator2/2  "Steering IF L Frc"
  Demux/17 -> Bus Creator2/1  "Steering IF SteerByTrq"
  Demux/16 -> Bus Creator1/16  "Steering IF R iSteer2q"
  Demux/15 -> Bus Creator1/15  "Steering IF R qpp"
  Demux/14 -> Bus Creator1/14  "Steering IF R qp"
  Demux/13 -> Bus Creator1/13  "Steering IF R q"
  Demux/12 -> Bus Creator1/12  "Steering IF L iSteer2q"
  Demux/11 -> Bus Creator1/11  "Steering IF L qpp"
  Demux/10 -> Bus Creator1/10  "Steering IF L qp"
  Demux/9 -> Bus Creator1/9  "Steering IF L q"
  Demux/8 -> Bus Creator1/8  "Steering IF AssistTrqPin"
  Demux/7 -> Bus Creator1/7  "Steering IF AssistTrqCol"
  Demux/6 -> Bus Creator1/6  "Steering IF AssistFrc"
  Demux/5 -> Bus Creator1/5  "Steering IF TrqStatic"
  Demux/4 -> Bus Creator1/4  "Steering IF Trq"
  Demux/3 -> Bus Creator1/3  "Steering IF AngAcc"
  Demux/2 -> Bus Creator1/2  "Steering IF AngVel"
  Demux/1 -> Bus Creator1/1  "Steering IF Ang"
  Bus Creator1/1 -> Steer.IF/1
  Steering/2 -> Demux/1
  Bus Creator2/1 -> Terminator/1  "Steer IF (in)"
  VhclCtrl.Steering/1 -> Steering/2
  Steering/1 -> Sync_Out/1
  Sync_In/1 -> Steering/1

== system CM13_2024a_MachE_for_UA_HIL/CarMaker_new/IPG Vehicle/CarAndTrailer/Trailer ==
  Sync_In : Inport
  Trailer.Load : Inport  Port=2
  Car.Hitch : Inport  Port=3
  Car.Fr1 : Inport  Port=4
  Car.Trq_T2W : Inport  Port=5
  WheelCarrier.Misc : Inport  Port=6
  CreateBus Car.Hitch.FrcTrq : Subsystem
  CreateBus Vhcl.Motion : Subsystem
  CreateBus Vhcl.PoI : Subsystem
  CreateBus Vhcl.Steering : Subsystem
  CreateBus Vhcl.Wheel.FL : Subsystem
  CreateBus Vhcl.Wheel.FR : Subsystem
  CreateBus Vhcl.Wheel.RL : Subsystem
  CreateBus Vhcl.Wheel.RR : Subsystem
  Trailer : S-Function  FunctionName=CM_Sfun  Parameters='Trailer'  SFunctionDeploymentMode=off  EnableBusSupport=off
  Sync_Out : Outport  VectorParamsAs1DForOutWhenUnconnected=off
  Vhcl.Steering : Outport  Port=2  VectorParamsAs1DForOutWhenUnconnected=off
  Vhcl.Motion : Outport  Port=3  VectorParamsAs1DForOutWhenUnconnected=off
  Vhcl.PoI : Outport  Port=4  VectorParamsAs1DForOutWhenUnconnected=off
  Vhcl.Wheel.FL : Outport  Port=5  VectorParamsAs1DForOutWhenUnconnected=off
  Vhcl.Wheel.FR : Outport  Port=6  VectorParamsAs1DForOutWhenUnconnected=off
  Vhcl.Wheel.RL : Outport  Port=7  VectorParamsAs1DForOutWhenUnconnected=off
  Vhcl.Wheel.RR : Outport  Port=8  VectorParamsAs1DForOutWhenUnconnected=off
  Car.Hitch.FrcTrq : Outport  Port=9  VectorParamsAs1DForOutWhenUnconnected=off
  wires:
  Trailer/2 -> CreateBus Vhcl.Steering/1(In1)
  CreateBus Vhcl.Steering/1(Out1) -> Vhcl.Steering/1  "Vhcl.Steering"
  Trailer/3 -> CreateBus Vhcl.Motion/1(In1)
  Trailer/4 -> CreateBus Vhcl.PoI/1(In1)
  Trailer/5 -> CreateBus Vhcl.Wheel.FL/1(In1)
  Trailer/6 -> CreateBus Vhcl.Wheel.FR/1(In1)
  Trailer/7 -> CreateBus Vhcl.Wheel.RL/1(In1)
  Trailer/9 -> CreateBus Car.Hitch.FrcTrq/1(In1)
  Trailer/8 -> CreateBus Vhcl.Wheel.RR/1(In1)
  CreateBus Vhcl.Wheel.RR/1(Out1) -> Vhcl.Wheel.RR/1  "Vhcl.Wheel.RR"
  CreateBus Vhcl.Wheel.RL/1(Out1) -> Vhcl.Wheel.RL/1  "Vhcl.Wheel.RL"
  CreateBus Vhcl.Wheel.FR/1(Out1) -> Vhcl.Wheel.FR/1  "Vhcl.Wheel.FR"
  CreateBus Vhcl.Wheel.FL/1(Out1) -> Vhcl.Wheel.FL/1  "Vhcl.Wheel.FL"
  CreateBus Vhcl.PoI/1(Out1) -> Vhcl.PoI/1  "Vhcl.PoI"
  CreateBus Vhcl.Motion/1(Out1) -> Vhcl.Motion/1  "Vhcl.Motion"
  Car.Trq_T2W/1 -> Trailer/5
  WheelCarrier.Misc/1 -> Trailer/6
  CreateBus Car.Hitch.FrcTrq/1(Out1) -> Car.Hitch.FrcTrq/1  "Car.Hitch.FrcTrq"
  Car.Fr1/1 -> Trailer/4
  Car.Hitch/1 -> Trailer/3
  Trailer.Load/1 -> Trailer/2
  Trailer/1 -> Sync_Out/1
  Sync_In/1 -> Trailer/1

== system CM13_2024a_MachE_for_UA_HIL/CarMaker_new/IPG Vehicle/Driver and Drive Cycle/Automation_Spd_selection ==
  note: Auther@MaxChen
  note: Note: Since all v_vut is assinged to init velocity,
      | we will use this number as the target testrun speed
  note: If CM reach postprocessing,
      | or vehicle has driven more than 150meter, set speed to 0
  note: TODO: This delay need to be larger. Maybe a real-time of 5 seconds
  note: If AEB flag is triggered, set speed to 0
      | If AEB flag is cleared:
      | 	if Master SW is ON, use TestRun File Speed Demond
      | 	else speed is 0
  AEB_IS_Triggered : Inport
  A_M_SW_sig : Inport  Port=2
  0_speed : Constant  Value=0
  Compare To Constant : simulink/Logic and Bit Operations/Compare To Constant  relop===  const=10  OutDataTypeStr=boolean
  Compare To Constant1 : simulink/Logic and Bit Operations/Compare To Constant  relop=>=  const=150  OutDataTypeStr=boolean
  Delay : Delay  DelayLength=5
  OR : Logic  Operator=OR  IconShape=distinctive  AllPortsSameDT=off  OutDataTypeStr=boolean
  Read CM Dict11 : CarMaker4SL/Read CM Dict  xname=Vhcl.Distance  xsync=off  xstime=Continuous
  Read CM Dict7 : CarMaker4SL/Read CM Dict  xname=SC.State  xsync=off  xstime=Continuous
  Read CM Parameter : CarMaker4SL/Read CM Parameter  xfile=Testrun  xkey=DrivMan.Init.Velocity  xnout=1  xdefaults=0  xmuxed=on  xstime=Continuous
      settings: SourceProductName=CarMaker4SL
  Switch : Switch  Criteria=u2 > Threshold  SaturateOnIntegerOverflow=off  InputSameDT=off
  Switch1 : Switch  Criteria=u2 > Threshold  SaturateOnIntegerOverflow=off  InputSameDT=off
  Switch2 : Switch  Criteria=u2 > Threshold  SaturateOnIntegerOverflow=off  InputSameDT=off
  Spd : Outport
  wires:
  AEB_IS_Triggered/1 -> Switch/2
  Switch/1 -> Switch2/3
  A_M_SW_sig/1 -> Delay/1
  0_speed/1 -> Switch1/3, Switch/1, Switch2/1
  Switch1/1 -> Switch/3
  Delay/1 -> Switch1/2
  Read CM Dict7/1 -> Compare To Constant/1  "SC.State"
  Compare To Constant/1 -> OR/2
  Switch2/1 -> Spd/1
  Read CM Parameter/1 -> Switch1/1  "v_vut"
  Read CM Dict11/1 -> Compare To Constant1/1  "Vhcl.Distance"
  Compare To Constant1/1 -> OR/1
  OR/1 -> Switch2/2

== system CM13_2024a_MachE_for_UA_HIL/CarMaker_new/IPG Vehicle/Driver and Drive Cycle/Driver and PI with FF Control ==
  Vehicle_Spd_kph : Inport
  Vehicle_SpdDmd_kph : Inport  Port=2
  Bus Creator : BusCreator  Inputs=6
  Constant : Constant
  Memory1 : Memory
  Memory2 : Memory
  SpdSat : Saturate  UpperLimit=190  LowerLimit=-5
  Vehicle Speed Controller : Subsystem
  km to miles : Gain  Gain=1/1.609344
  DriverBus : Outport
  wires:
  Vehicle Speed Controller/1(AcceleratorPedalPos) -> Bus Creator/2  "AccelPedalCmd"
  Vehicle_SpdDmd_kph/1 -> Memory1/1
  Constant/1 -> Bus Creator/1  "Drive"
  Vehicle Speed Controller/3(BrakeSwitch) -> Bus Creator/4
  SpdSat/1 -> Vehicle Speed Controller/1(RefSpd), km to miles/1, Bus Creator/5  "RefSpd [km/hr]"
  Vehicle Speed Controller/2(BrakePedalPos) -> Bus Creator/3  "BrakePedalCmd"
  Bus Creator/1 -> DriverBus/1  "DriverBus"
  Vehicle_Spd_kph/1 -> Memory2/1
  km to miles/1 -> Bus Creator/6  "RefSpd [mph]"
  Memory1/1 -> SpdSat/1
  Memory2/1 -> Vehicle Speed Controller/2(VehicleSpeed)
